simulink library "Pressure_Drop_PipeTheory"  (Simulink 8.2)
settings: Solver=ode45  StartTime=0.0  StopTime=10.0  RelTol=1e-3
undefined symbols (not defined in the file): DPConstant, DPLinear, DPQuadratic, Pressure
libraries: simulink x1, carnot x1
settings Model: Creator=drhf  LastModifiedBy=drhf

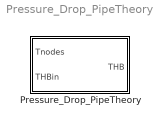
== system Pressure_Drop_PipeTheory ==
  Pressure_Drop_PipeTheory : Subsystem  mask(theoretical pressure drop of a pipe){dia=0.02, len=1, rough=0.04, nbend=1}
      mask prompts: dia "Diameter in m"; len "Length of pipe in m"; rough "Roughness of pipe in m"; nbend "Number of 90° bends"
      mask help: Calculates the pressure drop in a pipe according to a theoretical model.
      mask Help: web(fullfile(path_carnot('help'),'Pressure_Drop_PipeTheory.html'),'-helpbrowser')

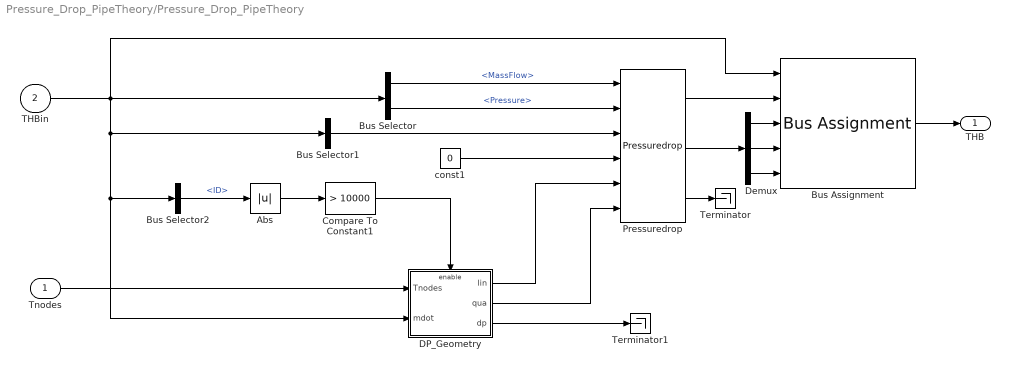
== system Pressure_Drop_PipeTheory/Pressure_Drop_PipeTheory ==
  Tnodes : Inport
  THBin : Inport  Port=2
  Abs : Abs
  Bus Assignment : BusAssignment  AssignedSignals=Pressure,DPConstant,DPLinear,DPQuadratic
  Bus Selector : BusSelector  OutputSignals=MassFlow,Pressure
  Bus Selector1 : BusSelector  OutputSignals=DPConstant,DPLinear,DPQuadratic  OutputAsBus=on
  Bus Selector2 : BusSelector  OutputSignals=ID
  Compare To Constant1 : simulink/Logic and Bit Operations/Compare To Constant  relop=>  const=10000  OutDataTypeStr=boolean
  DP_Geometry : Subsystem
  Demux : Demux  Outputs=3
  Pressuredrop : carnot/Basic/Pressure_Drop/Pressuredrop
  Terminator : Terminator
  Terminator1 : Terminator
  const1 : Constant  Value=0
  THB : Outport
  wires:
  const1/1 -> Pressuredrop/4
  Pressuredrop/3 -> Terminator/1
  Compare To Constant1/1 -> DP_Geometry/Enable
  Tnodes/1 -> DP_Geometry/1(Tnodes)
  Bus Selector2/1 -> Abs/1  "<ID>"
  Bus Selector/2 -> Pressuredrop/2  "<Pressure>"
  Bus Selector/1 -> Pressuredrop/1  "<MassFlow>"
  Bus Selector1/1 -> Pressuredrop/3
  Abs/1 -> Compare To Constant1/1
  THBin/1 -> Bus Assignment/1, DP_Geometry/2(mdot), Bus Selector2/1, Bus Selector1/1, Bus Selector/1
  Bus Assignment/1 -> THB/1
  Pressuredrop/1 -> Bus Assignment/2
  Demux/1 -> Bus Assignment/3
  Demux/2 -> Bus Assignment/4
  Demux/3 -> Bus Assignment/5
  Pressuredrop/2 -> Demux/1
  DP_Geometry/1(lin) -> Pressuredrop/5
  DP_Geometry/2(qua) -> Pressuredrop/6
  DP_Geometry/3(dp) -> Terminator1/1

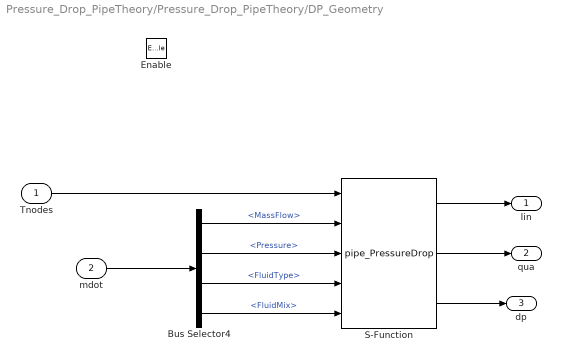
== system Pressure_Drop_PipeTheory/Pressure_Drop_PipeTheory/DP_Geometry ==
  Tnodes : Inport
  mdot : Inport  Port=2
  Enable : EnablePort
  Bus Selector4 : BusSelector  OutputSignals=MassFlow,Pressure,FluidType,FluidMix
  S-Function : S-Function  FunctionName=pipe_PressureDrop  Parameters="dia, len,  rough, nbend"  EnableBusSupport=off
  lin : Outport  OutputWhenDisabled=reset  InitialOutput=0
  qua : Outport  Port=2  OutputWhenDisabled=reset  InitialOutput=0
  dp : Outport  Port=3  OutputWhenDisabled=reset  InitialOutput=0
  wires:
  S-Function/3 -> dp/1
  Bus Selector4/4 -> S-Function/5  "<FluidMix>"
  Bus Selector4/3 -> S-Function/4  "<FluidType>"
  Bus Selector4/2 -> S-Function/3  "<Pressure>"
  Bus Selector4/1 -> S-Function/2  "<MassFlow>"
  mdot/1 -> Bus Selector4/1
  S-Function/2 -> qua/1
  S-Function/1 -> lin/1
  Tnodes/1 -> S-Function/1
